simulink model "untitled"  (R2019a)
settings: Solver=VariableStepAuto  StartTime=0.0  StopTime=10.0  RelTol=1e-3
settings Model: Creator=hxl0tp5  LastModifiedBy=hxl0tp5

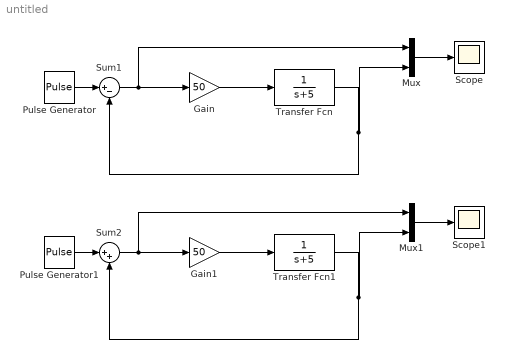
== system untitled ==
  Gain : Gain  Gain=50
  Gain1 : Gain  Gain=50
  Mux : Mux  Inputs=2
  Mux1 : Mux  Inputs=2
  Pulse Generator : DiscretePulseGenerator  PulseType=Time based  Period=10  PulseWidth=5
  Pulse Generator1 : DiscretePulseGenerator  PulseType=Time based  Period=10  PulseWidth=5
  Scope : Scope
  Scope1 : Scope
  Sum1 : Sum  Inputs=|+-
  Sum2 : Sum  Inputs=|++
  Transfer Fcn : TransferFcn  Denominator=[1 5]
  Transfer Fcn1 : TransferFcn  Denominator=[1 5]
  wires:
  Pulse Generator/1 -> Sum1/1
  Transfer Fcn/1 -> Mux/2, Sum1/2
  Sum1/1 -> Gain/1, Mux/1
  Gain/1 -> Transfer Fcn/1
  Mux/1 -> Scope/1
  Transfer Fcn1/1 -> Mux1/2, Sum2/2
  Gain1/1 -> Transfer Fcn1/1
  Sum2/1 -> Gain1/1, Mux1/1
  Pulse Generator1/1 -> Sum2/1
  Mux1/1 -> Scope1/1
